simulink model "Koopman_lMPC"  (R2022b)
settings: Solver=FixedStepAuto  StartTime=0.0  StopTime=Tf  FixedStep=Ts  RelTol=1e-3
values from neighbouring files (symbols this model uses):
  A_EKF = A(1:n_x,:)    [vdp_MPC.m]
  B_EKF = B(1:n_x,:)    [vdp_MPC.m]
  C_EKF = C    [vdp_MPC.m]
  eta = 0.001    [vdp_MPC.m]
  S0_EKF = Spline_Radial_Obs([0;0], X0)    [vdp_MPC.m]
  Ts = 0.01    [EKF_Koopman.m]    (also in scope_plotting.m)
undefined symbols (not defined in the file or in its folder): DiscIntNeverNeededParam
libraries: mpclib x1
settings Model: Creator=sergiovaneg  LastModifiedBy=sergiovaneg
settings ModelReferenceCC: EnableRefExpFcnMdlSchedulingChecks=on

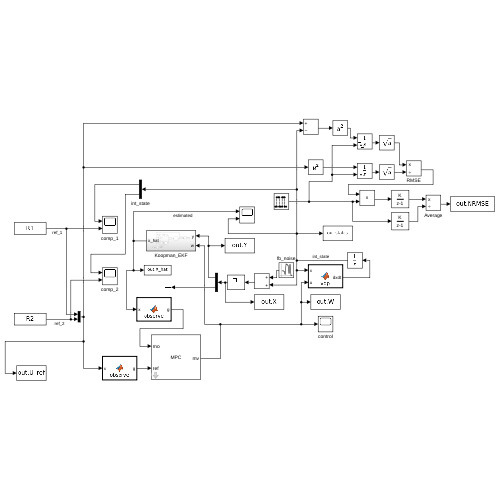
[thumbnail: Simulink's stored preview of the top-level diagram]
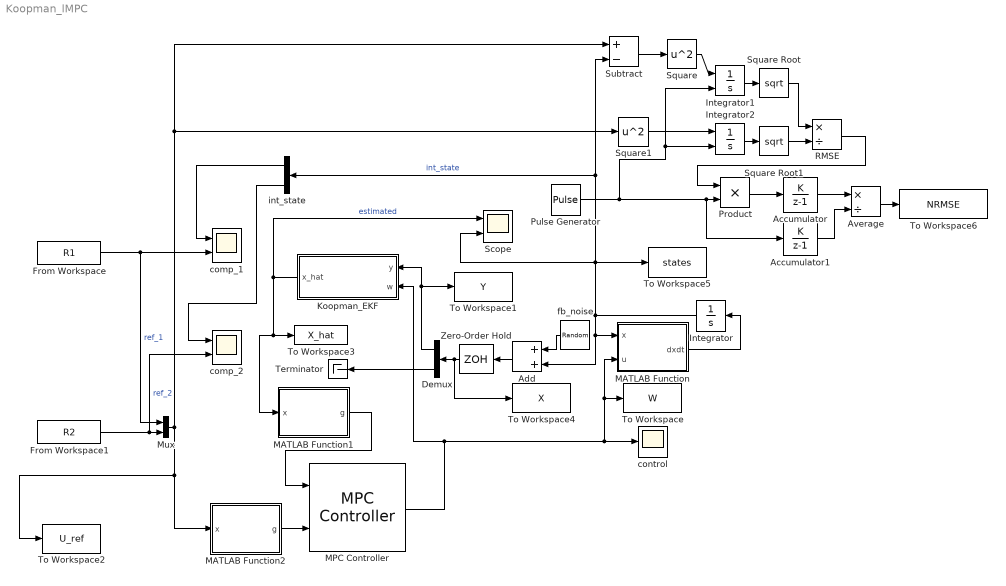
== system Koopman_lMPC ==
  Accumulator : DiscreteIntegrator  IntegratorMethod=Accumulation: Forward Euler  InitialCondition=[0;0]  SampleTime=Ts  ICPrevOutput=DiscIntNeverNeededParam  ICPrevScaledInput=DiscIntNeverNeededParam
  Accumulator1 : DiscreteIntegrator  IntegratorMethod=Accumulation: Forward Euler  SampleTime=-1  ICPrevOutput=DiscIntNeverNeededParam  ICPrevScaledInput=DiscIntNeverNeededParam
  Add : Sum
  Average : Product  Inputs=*/
  Demux : Demux  Outputs=2
  From Workspace : FromWorkspace  VariableName=R1
  From Workspace1 : FromWorkspace  VariableName=R2
  Integrator : Integrator  InitialCondition=[0;0]
  Integrator1 : Integrator  ExternalReset=falling  InitialCondition=[0;0]
  Integrator2 : Integrator  ExternalReset=falling  InitialCondition=[eps;eps]
  Koopman_EKF : Subsystem
  MATLAB Function : MATLAB Function  TreatAsAtomicUnit=on
  MATLAB Function1 : MATLAB Function  TreatAsAtomicUnit=on
  MATLAB Function2 : MATLAB Function  TreatAsAtomicUnit=on
  MPC Controller : mpclib/MPC Controller  SCDEnableBlockLinearizationSpecification=on  mpcobj=controller  x0=ctrl_0  is_multiple=0  enable_value=0  return_u0=off  updateMPCinCallerWorkspace=on  md_inport=off  mv_inport=off  uref_inport=off  return_cost=off  return_mvseq=off  return_qpstatus=off  return_xseq=off  return_state=off  return_ovseq=off  state_inport=off  umin_inport=off  umax_inport=off  ymin_inport=off  ymax_inport=off  cc_inport=off  ywt_inport=off  uwt_inport=off  duwt_inport=off  rhoeps_inport=off  pm_inport=off  MaximumP=10  HorizonChoice=FixedHorizon  n_ts=0.01  n_p=25  n_mv=1  n_md=0  n_ud=0  n_mo=77  n_uo=0  BlockDataType=double  SampleTimeInherited=off  switch_inport=off
  Mux : Mux  Inputs=2
  Product : Product
  Pulse Generator : DiscretePulseGenerator  Period=10/Ts  SampleTime=Ts
  RMSE : Product  Inputs=*/
  Scope : Scope  NumInputPorts=2
  Square : Math  Operator=square
  Square Root : Sqrt
  Square Root1 : Sqrt
  Square1 : Math  Operator=square
  Subtract : Sum  Inputs=+-
  Terminator : Terminator
  To Workspace : ToWorkspace  VariableName=W  SampleTime=Ts
      settings: Save2DSignal=2-D array (concatenate along first dimension)
  To Workspace1 : ToWorkspace  VariableName=Y  SampleTime=Ts
      settings: Save2DSignal=2-D array (concatenate along first dimension)
  To Workspace2 : ToWorkspace  VariableName=U_ref  SampleTime=Ts
      settings: Save2DSignal=2-D array (concatenate along first dimension)
  To Workspace3 : ToWorkspace  VariableName=X_hat  SampleTime=Ts
      settings: Save2DSignal=2-D array (concatenate along first dimension)
  To Workspace4 : ToWorkspace  VariableName=X  SampleTime=Ts
      settings: Save2DSignal=2-D array (concatenate along first dimension)
  To Workspace5 : ToWorkspace  VariableName=states  SampleTime=Ts
      settings: Save2DSignal=2-D array (concatenate along first dimension)
  To Workspace6 : ToWorkspace  VariableName=NRMSE  SampleTime=-1
      settings: MaxDataPoints=1  Save2DSignal=2-D array (concatenate along first dimension)
  Zero-Order Hold : ZeroOrderHold  SampleTime=Ts
  comp_1 : Scope  NumInputPorts=2
  comp_2 : Scope  NumInputPorts=2
  control : Scope
  fb_noise : RandomNumber  Variance=eta  Seed=[2;3]  SampleTime=Ts
  int_state : Demux  Outputs=2
  wires:
  int_state/1 -> comp_1/1
  fb_noise/1 -> Add/1
  MPC Controller/1 -> Koopman_EKF/2(w), MATLAB Function/2(u), To Workspace/1, control/1
  Integrator/1 -> Subtract/2, int_state/1, Scope/2, To Workspace5/1, Add/2, MATLAB Function/1(x)  "int_state"
  From Workspace1/1 -> comp_2/2, Mux/2  "ref_2"
  int_state/2 -> comp_2/1
  MATLAB Function/1(dxdt) -> Integrator/1
  Mux/1 -> To Workspace2/1, MATLAB Function2/1(x), Subtract/1, Square1/1
  Demux/1 -> Koopman_EKF/1(y), To Workspace1/1
  Demux/2 -> Terminator/1
  Koopman_EKF/1(x_hat) -> MATLAB Function1/1(x), To Workspace3/1, Scope/1  "estimated"
  Zero-Order Hold/1 -> To Workspace4/1, Demux/1
  Add/1 -> Zero-Order Hold/1
  Subtract/1 -> Square/1
  Square/1 -> Integrator1/1
  From Workspace/1 -> comp_1/2, Mux/1  "ref_1"
  Integrator1/1 -> Square Root/1
  MATLAB Function1/1(g) -> MPC Controller/1
  MATLAB Function2/1(g) -> MPC Controller/2
  Square Root/1 -> RMSE/1
  Integrator2/1 -> Square Root1/1
  Square1/1 -> Integrator2/1
  Square Root1/1 -> RMSE/2
  Pulse Generator/1 -> Accumulator1/1, Product/2, Integrator1/2, Integrator2/2
  Accumulator/1 -> Average/1
  Product/1 -> Accumulator/1
  RMSE/1 -> Product/1
  Accumulator1/1 -> Average/2
  Average/1 -> To Workspace6/1

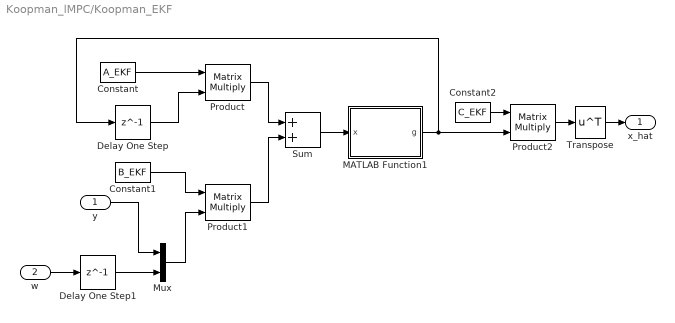
== system Koopman_lMPC/Koopman_EKF ==
  y : Inport
  w : Inport  Port=2
  Constant : Constant  Value=A_EKF
  Constant1 : Constant  Value=B_EKF
  Constant2 : Constant  Value=C_EKF
  Delay One Step : Delay  DelayLength=1  InitialCondition=S0_EKF
  Delay One Step1 : Delay  DelayLength=1  InitialCondition=0
  MATLAB Function1 : MATLAB Function  TreatAsAtomicUnit=on
  Mux : Mux  Inputs=2
  Product : Product  Multiplication=Matrix(*)
  Product1 : Product  Multiplication=Matrix(*)
  Product2 : Product  Multiplication=Matrix(*)
  Sum : Sum
  Transpose : Math  Operator=transpose
  x_hat : Outport
  wires:
  Constant/1 -> Product/1
  Delay One Step/1 -> Product/2
  Product/1 -> Sum/1
  Constant1/1 -> Product1/1
  Product1/1 -> Sum/2
  Sum/1 -> MATLAB Function1/1(x)
  Constant2/1 -> Product2/1
  w/1 -> Delay One Step1/1
  y/1 -> Mux/1
  Mux/1 -> Product1/2
  Delay One Step1/1 -> Mux/2
  MATLAB Function1/1(g) -> Product2/2, Delay One Step/1
  Product2/1 -> Transpose/1
  Transpose/1 -> x_hat/1

== matlab function Koopman_lMPC/MATLAB Function ==
  data: x input; u input; dxdt output
function dxdt = vdp(x,u)
    dxdt = zeros(2,1);
    dxdt(1) = 2*x(2);
    dxdt(2) = -0.8*x(1)+2*x(2)-10*(x(1)^2)*x(2)+u;

== matlab function Koopman_lMPC/MATLAB Function1 ==
  data: x input; g output; X0_VDP parameter
function g = observe(x,X0_VDP)
    g=zeros(size(x,1)+size(X0_VDP,2),1);
    aux = vecnorm(X0_VDP-x)';
    g(1:size(x,1))=x;
    g(size(x,1)+1:end)=aux.*log(aux.^aux);
end

== matlab function Koopman_lMPC/MATLAB Function2 ==
  data: x input; g output; X0_VDP parameter
function g = observe(x,X0_VDP)
    g=zeros(size(x,1)+size(X0_VDP,2),1);
    aux = vecnorm(X0_VDP-x)';
    g(1:size(x,1))=x;
    g(size(x,1)+1:end)=aux.*log(aux.^aux);
end

== matlab function Koopman_lMPC/Koopman_EKF/MATLAB Function1 ==
  data: x input; g output; X0_EKF parameter
function g = observe(x,X0_EKF)
    g=zeros(size(x,1)+size(X0_EKF,2),1);
    aux = vecnorm(X0_EKF-x)';
    g(1:size(x,1))=x;
    g(size(x,1)+1:end)=aux.*log(aux.^aux);
end
